simulink library "simeventsgates1"  (Simulink 7.4)
settings: Solver=ode45  SolverMode=SingleTasking  StartTime=0.0  StopTime=10.0  RelTol=1e-3
undefined symbols (not defined in the file or in its folder): des_support, gcbh
libraries: des_sfun_lib x2
settings Model: ForwardingTableString=||__slOldName__||simeventsgates1/Signal Latch||__slNewName__||simeventssignalmanage1/Signal Latch  Creator=mclune  LastModifiedBy=frodin  ExtModeAutoUpdateStatusClock=off

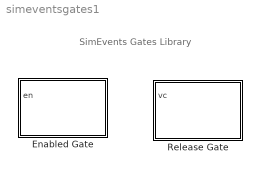
== system simeventsgates1 ==
  note: SimEvents Gates Library
  Enabled Gate : Subsystem  Priority=1  LoadFcn=des_support('desLoadFcn',gcbh)  StartFcn=des_support('desStartFcn',gcbh)  StopFcn=des_support('desStopFcn',gcbh)  mask(Enabled Gate){SpecifyEventPriority=off, PriorityGateEnableOpenClose=2000, StatNumberDeparted=Off}
      mask prompts: SpecifyEventPriority "Resolve simultaneous signal updates according to event priority"; PriorityGateEnableOpenClose "Event priority:"; StatNumberDeparted "Number of entities departed, #d:"
      mask help:
      | Allow or forbid entity arrivals based on an enable signal. The entity input port is available for entity arrivals if the control signal is positive.
      | Arriving entities depart immediately.
      mask init:
      | des_enabled_gatemask(gcb, 'init','apply')
      settings: CopyFcn=des_support('desCopyFcn',gcbh)  DeleteFcn=des_support('desDeleteFcn',gcbh)  UndoDeleteFcn=des_support('desUndoDeleteFcn',gcbh)  ModelCloseFcn=des_support('desModelCloseFcn',gcbh)  PreSaveFcn=des_support('desPreSaveFcn',gcbh)  PostSaveFcn=des_support('desPostSaveFcn',gcbh)  NameChangeFcn=des_support('desNameChangeFcn',gcbh)  CloseFcn=des_support('desCloseFcn',gcbh)  ErrorFcn=des_error_redirect
      mask Help: helpview(simeventsbhelp)
      mask StyleString: checkbox,edit,popup(Off|On|Upon stop or pause)
      mask CallbackString: des_enabled_gatemask(gcb,'cbSpecifyEventPriority','noapply');||des_enabled_gatemask(gcb,'cbStatNumberDeparted','noapply');
      mask TabNameString: Enabled Gate,Enabled Gate,Statistics
      mask Display:
      | image(des_iconLoad('gatesEnable.jpg'),'center');
      | port_label('LConn',1,'IN');
      | port_label('input',1,'en');
      | port_label('RConn',1,'OUT');
  Release Gate : Subsystem  Priority=1  LoadFcn=des_support('desLoadFcn',gcbh)  StartFcn=des_support('desStartFcn',gcbh)  StopFcn=des_support('desStopFcn',gcbh)  mask(Release Gate){OpenGateUpon=Change in signal from port vc, SignalEdgeOption=Rising, SpecifyEventPriority=off, PriorityGateRelease=2200, StatNumberDeparted=Off}
      mask prompts: OpenGateUpon "Open gate upon:"; SignalEdgeOption "Type of change in signal value:"; SpecifyEventPriority "Resolve simultaneous signal updates according to event priority"; PriorityGateRelease "Event priority:"; StatNumberDeparted "Number of entities departed, #d:"
      mask help: Open the gate to permit at most one pending entity to advance and then close the gate immediately. The Open gate upon parameter indicates the type of event that causes the gate to open.
      mask init:
      | des_releasegatemask(gcb, 'init','apply')
      settings: CopyFcn=des_support('desCopyFcn',gcbh)  DeleteFcn=des_support('desDeleteFcn',gcbh)  UndoDeleteFcn=des_support('desUndoDeleteFcn',gcbh)  ModelCloseFcn=des_support('desModelCloseFcn',gcbh)  PreSaveFcn=des_support('desPreSaveFcn',gcbh)  PostSaveFcn=des_support('desPostSaveFcn',gcbh)  NameChangeFcn=des_support('desNameChangeFcn',gcbh)  CloseFcn=des_support('desCloseFcn',gcbh)  ErrorFcn=des_error_redirect
      mask Help: helpview(simeventsbhelp)
      mask StyleString: popup(Sample time hit from port ts|Trigger from port tr|Change in signal from port vc|Function call from port fcn),popup(Rising|Falling|Either),checkbox,edit,popup(Off|On|Upon stop or pause)
      mask CallbackString: des_releasegatemask(gcb,'cbOpenGateUpon','noapply');|des_releasegatemask(gcb,'cbSignalEdgeOption','noapply');|des_releasegatemask(gcb,'cbSpecifyEventPriority','noapply');||des_releasegatemask(gcb,'cbStatNumberDeparted','noapply');
      mask TabNameString: Release Gate,Release Gate,Release Gate,Release Gate,Statistics
      mask Display:
      | image(des_iconLoad('gatesRelease.jpg'),'center');
      | port_label('LConn',1,'IN');
      | port_label('input',1,'vc');
      | port_label('RConn',1,'OUT');

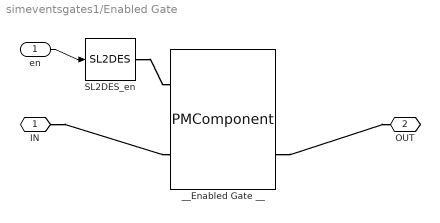
== system simeventsgates1/Enabled Gate ==
  en : Inport  PortDimensions=1  DataType=double  OutDataType=sfix(16)  OutScaling=2^0  OutDataTypeStr=double
  SL2DES_en : des_sfun_lib/SL2DES  SystemSampleTime=-1  PortType=desPortOut  PhysicalDomain=simevents  SubClassName=DES_SL2DES  timingControl=Simulink  execIndex=1  trigger=None  filter=0  updateBeforeRead=off  InitValue=0  initToFactVal=off  sampleTime=-1  offsetTime=0  idxBlockMR=0  IsMonitorOnly=off  dimsInfo=1
  __Enabled Gate __ : PMComponent  PhysicalDomain=simevents  SubClassName=DES_ENABLED_GATE  LeftPortType=desPortIn  RightPortType=desPortOut  LConnTagsString=DI|DI  RConnTagsString=DO|DO
      mask Display:
      | port_label('LConn',1,'en');
      | port_label('LConn',2,'IN');
      | port_label('RConn',1,'#d');
      | port_label('RConn',2,'OUT');
  IN : PMIOPort  Port=1  Side=Left
  OUT : PMIOPort  Port=2  Side=Right
  wires:
  en/1 -> SL2DES_en/1
  connections:
  IN/RConn1 -- __Enabled Gate __/LConn2
  __Enabled Gate __/RConn2 -- OUT/RConn1
  SL2DES_en/RConn1 -- __Enabled Gate __/LConn1

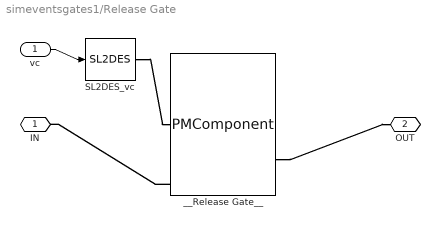
== system simeventsgates1/Release Gate ==
  vc : Inport  PortDimensions=1  DataType=double  OutDataType=sfix(16)  OutScaling=2^0  OutDataTypeStr=double
  SL2DES_vc : des_sfun_lib/SL2DES  SystemSampleTime=-1  PortType=desPortOut  PhysicalDomain=simevents  SubClassName=DES_SL2DES  timingControl=Simulink  execIndex=2200  trigger=None  filter=0  updateBeforeRead=off  InitValue=0  initToFactVal=off  sampleTime=-1  offsetTime=0  idxBlockMR=0  IsMonitorOnly=off  dimsInfo=1
  __Release Gate__ : PMComponent  PhysicalDomain=simevents  SubClassName=DES_RELEASE_GATE  LeftPortType=desPortIn  RightPortType=desPortOut  LConnTagsString=DI|DI|DI|DI|DI  RConnTagsString=DO|DO
      mask Display:
      | port_label('LConn',1,'ts');
      | port_label('LConn',2,'tr');
      | port_label('LConn',3,'vc');
      | port_label('LConn',4,'fcn');
      | port_label('LConn',5,'IN');
      | port_label('RConn',1,'#d');
      | port_label('RConn',2,'OUT');
  IN : PMIOPort  Port=1  Side=Left
  OUT : PMIOPort  Port=2  Side=Right
  wires:
  vc/1 -> SL2DES_vc/1
  connections:
  SL2DES_vc/RConn1 -- __Release Gate__/LConn3
  __Release Gate__/RConn2 -- OUT/RConn1
  __Release Gate__/LConn5 -- IN/RConn1
